simulink model "Polinomoal"  (Simulink 7.9)
settings: Solver=ode45  StartTime=0.0  StopTime=10.0  RelTol=1e-3
libraries: simulink x3
settings Model: Creator=Mihail  LastModifiedBy=Mihail

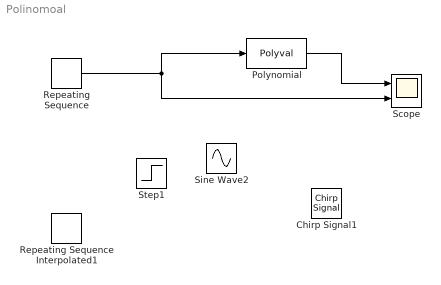
== system Polinomoal ==
  Chirp Signal1 : simulink/Sources/Chirp Signal  f1=0.1  T=100  f2=1
  Polynomial : Polyval  Coefs=[ +2, 1, 5,-8 ]
  Repeating Sequence : simulink/Sources/Repeating Sequence  rep_seq_t=[0 2]  rep_seq_y=[0 2]
  Repeating Sequence Interpolated1 : simulink/Sources/Repeating Sequence Interpolated  OutValues=[3 1 4 2 1].'  TimeValues=[0 0.1 0.5 0.6 1].'  LookUpMeth=Interpolation-Use End Values  tsamp=0.01  OutMin=[]  OutMax=[]  OutDataTypeStr=double  OutputDataTypeScalingMode=double  OutDataType=fixdt(0,8)  OutScaling=2^-10
  Scope : Scope  NumInputPorts=2
      settings: YMin=-5~-5  YMax=5~5
  Sine Wave2 : Sin  SampleTime=0
  Step1 : Step  SampleTime=0
  wires:
  Polynomial/1 -> Scope/1
  Repeating Sequence/1 -> Polynomial/1, Scope/2
